simulink model "ROBOT_MODEL_5_OTT"  (R2020a)
settings: Solver=FixedStepAuto  StartTime=0.0  StopTime=3  FixedStep=0.0001  RelTol=1e-3
values from neighbouring files (symbols this model uses):
  g = 9.81    [fast_init.m]
  I1 = 1    [fast_init.m]
  I2 = 10    [fast_init.m]
  ini_theta1 = 0    [fast_init.m]
  ini_theta1_d = 0    [fast_init.m]
  ini_theta2 = 0    [fast_init.m]
  ini_theta2_d = 0    [fast_init.m]
  ini_x1 = ini_x0+r1*cos(pi/2 - ini_theta1)    [fast_init.m]
  ini_x1_d = 0    [fast_init.m]
  ini_x2 = ini_xH + r2*cos(pi/2 - ini_theta2)    [fast_init.m]
  ini_x2_d = 0    [fast_init.m]
  ini_y1 = ini_y0+r1*sin(pi/2 - ini_theta1)    [fast_init.m]
  ini_y1_d = 0    [fast_init.m]
  M1 = 1    [fast_init.m]
  M2 = 10    [fast_init.m]
  r1 = 0.5    [fast_init.m]
  r2 = 0.4    [fast_init.m]
settings Model: Creator=fabia  LastModifiedBy=mic-ciciolla

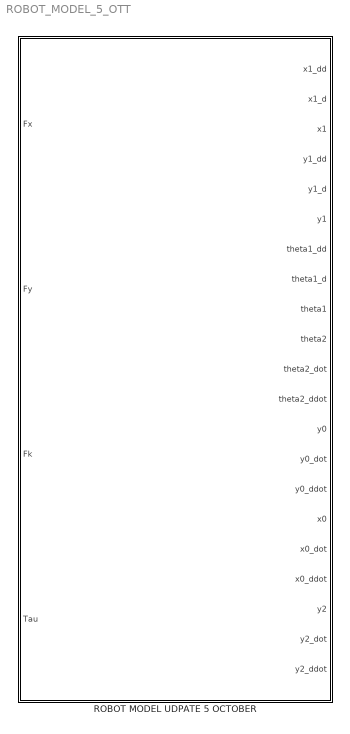
== system ROBOT_MODEL_5_OTT ==
  " ROBOT MODEL UDPATE 5 OCTOBER " : Subsystem

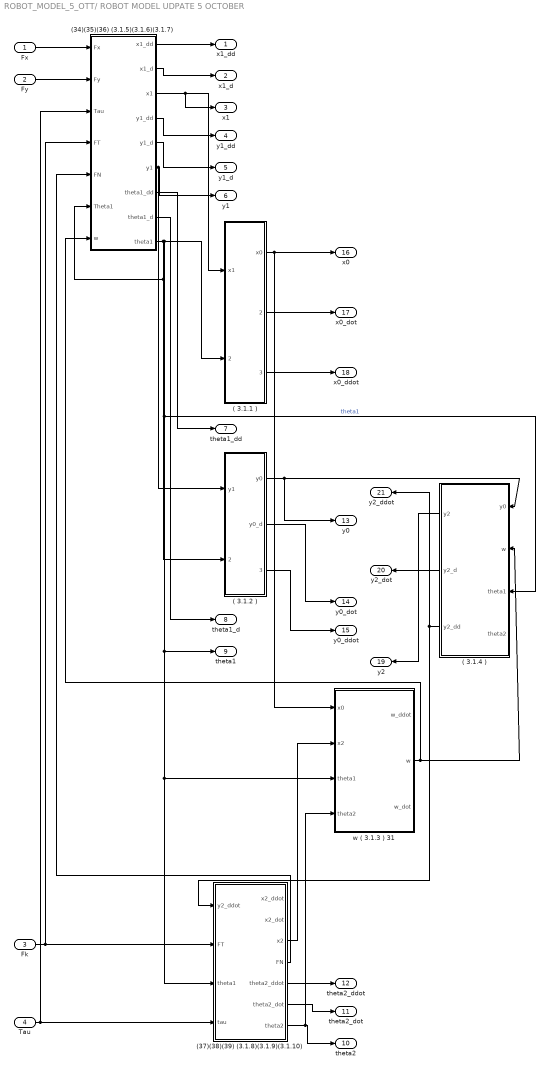
== system ROBOT_MODEL_5_OTT/ ROBOT MODEL UDPATE 5 OCTOBER  ==
  Fx : Inport
  Fy : Inport  Port=2
  Fk : Inport  Port=3
  Tau : Inport  Port=4
  "( 3.1.1 ) " : Subsystem
  ( 3.1.2 ) : Subsystem
  ( 3.1.4 ) : Subsystem
  (34)(35)(36) (3.1.5)(3.1.6)(3.1.7) : Subsystem
  (37)(38)(39) (3.1.8)(3.1.9)(3.1.10) : Subsystem
  w ( 3.1.3 ) 31 : Subsystem
  x1_dd : Outport
  x1_d : Outport  Port=2
  x1 : Outport  Port=3
  y1_dd : Outport  Port=4
  y1_d : Outport  Port=5
  y1 : Outport  Port=6
  theta1_dd : Outport  Port=7
  theta1_d : Outport  Port=8
  theta1 : Outport  Port=9
  theta2 : Outport  Port=10
  theta2_dot : Outport  Port=11
  theta2_ddot : Outport  Port=12
  y0 : Outport  Port=13
  y0_dot : Outport  Port=14
  y0_ddot : Outport  Port=15
  x0 : Outport  Port=16
  x0_dot : Outport  Port=17
  x0_ddot : Outport  Port=18
  y2 : Outport  Port=19
  y2_dot : Outport  Port=20
  y2_ddot : Outport  Port=21
  wires:
  ( 3.1.2 )/1(y0) -> ( 3.1.4 )/1(y0), y0/1
  "( 3.1.1 ) "/1(x0) -> w ( 3.1.3 ) 31/1(x0), x0/1
  ( 3.1.4 )/3(y2_dd) -> (37)(38)(39) (3.1.8)(3.1.9)(3.1.10)/1(y2_ddot), y2_ddot/1
  (34)(35)(36) (3.1.5)(3.1.6)(3.1.7)/3(x1) -> "( 3.1.1 ) "/1(x1), x1/1
  ( 3.1.4 )/2(y2_d) -> y2_dot/1
  (34)(35)(36) (3.1.5)(3.1.6)(3.1.7)/4(y1_dd) -> y1_dd/1
  ( 3.1.2 )/3(y0_dd) -> y0_ddot/1
  (37)(38)(39) (3.1.8)(3.1.9)(3.1.10)/3(x2) -> w ( 3.1.3 ) 31/2(x2)
  (37)(38)(39) (3.1.8)(3.1.9)(3.1.10)/4(FN) -> (34)(35)(36) (3.1.5)(3.1.6)(3.1.7)/5(FN)
  (34)(35)(36) (3.1.5)(3.1.6)(3.1.7)/1(x1_dd) -> x1_dd/1
  (37)(38)(39) (3.1.8)(3.1.9)(3.1.10)/5(theta2_ddot) -> theta2_ddot/1
  w ( 3.1.3 ) 31/2(w) -> ( 3.1.4 )/2(w), (34)(35)(36) (3.1.5)(3.1.6)(3.1.7)/7(w)
  (37)(38)(39) (3.1.8)(3.1.9)(3.1.10)/6(theta2_dot) -> theta2_dot/1
  Fy/1 -> (34)(35)(36) (3.1.5)(3.1.6)(3.1.7)/2(Fy)
  ( 3.1.4 )/1(y2) -> y2/1
  (37)(38)(39) (3.1.8)(3.1.9)(3.1.10)/7(theta2) -> w ( 3.1.3 ) 31/4(theta2), theta2/1
  (34)(35)(36) (3.1.5)(3.1.6)(3.1.7)/7(theta1_dd) -> theta1_dd/1
  Fx/1 -> (34)(35)(36) (3.1.5)(3.1.6)(3.1.7)/1(Fx)
  (34)(35)(36) (3.1.5)(3.1.6)(3.1.7)/2(x1_d) -> x1_d/1
  "( 3.1.1 ) "/2(x0_dot) -> x0_dot/1
  ( 3.1.2 )/2(y0_d) -> y0_dot/1
  Tau/1 -> (34)(35)(36) (3.1.5)(3.1.6)(3.1.7)/3(Tau), (37)(38)(39) (3.1.8)(3.1.9)(3.1.10)/4(tau)
  (34)(35)(36) (3.1.5)(3.1.6)(3.1.7)/8(theta1_d) -> theta1_d/1
  (34)(35)(36) (3.1.5)(3.1.6)(3.1.7)/5(y1_d) -> y1_d/1
  "( 3.1.1 ) "/3(x0_ddot) -> x0_ddot/1
  (34)(35)(36) (3.1.5)(3.1.6)(3.1.7)/6(y1) -> ( 3.1.2 )/1(y1), y1/1
  (34)(35)(36) (3.1.5)(3.1.6)(3.1.7)/9(theta1) -> ( 3.1.2 )/2(theta1), (34)(35)(36) (3.1.5)(3.1.6)(3.1.7)/6(Theta1), (37)(38)(39) (3.1.8)(3.1.9)(3.1.10)/3(theta1), w ( 3.1.3 ) 31/3(theta1), theta1/1, ( 3.1.4 )/3(theta1), "( 3.1.1 ) "/2(theta1)  "theta1"
  Fk/1 -> (34)(35)(36) (3.1.5)(3.1.6)(3.1.7)/4(FT), (37)(38)(39) (3.1.8)(3.1.9)(3.1.10)/2(FT)

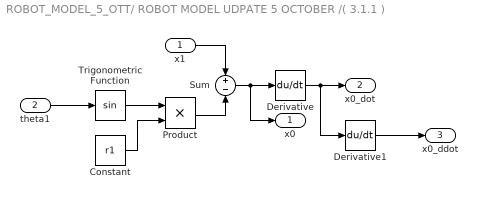
== system ROBOT_MODEL_5_OTT/ ROBOT MODEL UDPATE 5 OCTOBER /( 3.1.1 )  ==
  x1 : Inport
  theta1 : Inport  Port=2
  Constant : Constant  Value=r1
  Derivative : Derivative
  Derivative1 : Derivative
  Product : Product
  Sum : Sum  Inputs=+-
  Trigonometric Function : Trigonometry
  x0 : Outport
  x0_dot : Outport  Port=2
  x0_ddot : Outport  Port=3
  wires:
  Sum/1 -> x0/1, Derivative/1
  Derivative/1 -> x0_dot/1, Derivative1/1
  theta1/1 -> Trigonometric Function/1
  Trigonometric Function/1 -> Product/1
  x1/1 -> Sum/1
  Product/1 -> Sum/2
  Derivative1/1 -> x0_ddot/1
  Constant/1 -> Product/2

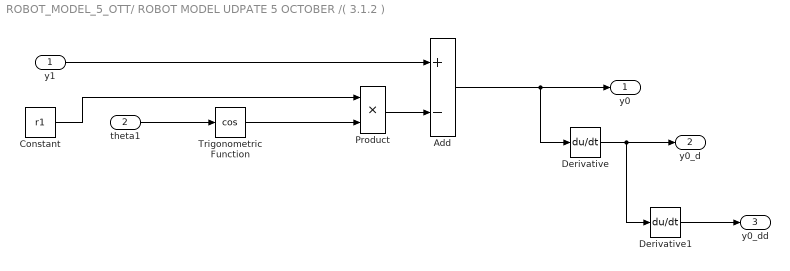
== system ROBOT_MODEL_5_OTT/ ROBOT MODEL UDPATE 5 OCTOBER /( 3.1.2 ) ==
  y1 : Inport
  theta1 : Inport  Port=2
  Add : Sum  Inputs=+-
  Constant : Constant  Value=r1
  Derivative : Derivative
  Derivative1 : Derivative
  Product : Product
  Trigonometric Function : Trigonometry  Operator=cos
  y0 : Outport
  y0_d : Outport  Port=2
  y0_dd : Outport  Port=3
  wires:
  y1/1 -> Add/1
  theta1/1 -> Trigonometric Function/1
  Trigonometric Function/1 -> Product/2
  Add/1 -> Derivative/1, y0/1
  Derivative/1 -> y0_d/1, Derivative1/1
  Derivative1/1 -> y0_dd/1
  Product/1 -> Add/2
  Constant/1 -> Product/1

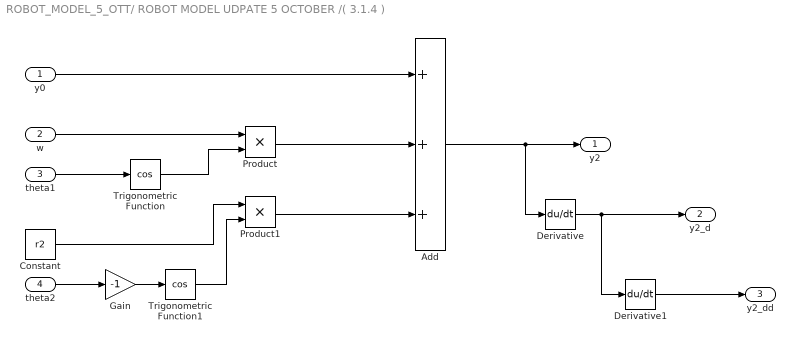
== system ROBOT_MODEL_5_OTT/ ROBOT MODEL UDPATE 5 OCTOBER /( 3.1.4 ) ==
  y0 : Inport
  w : Inport  Port=2
  theta1 : Inport  Port=3
  theta2 : Inport  Port=4
  Add : Sum  Inputs=+++
  Constant : Constant  Value=r2
  Derivative : Derivative
  Derivative1 : Derivative
  Gain : Gain  Gain=-1
  Product : Product
  Product1 : Product
  Trigonometric Function : Trigonometry  Operator=cos
  Trigonometric Function1 : Trigonometry  Operator=cos
  y2 : Outport
  y2_d : Outport  Port=2
  y2_dd : Outport  Port=3
  wires:
  y0/1 -> Add/1
  theta1/1 -> Trigonometric Function/1
  w/1 -> Product/1
  Trigonometric Function/1 -> Product/2
  Product/1 -> Add/2
  theta2/1 -> Gain/1
  Gain/1 -> Trigonometric Function1/1
  Trigonometric Function1/1 -> Product1/2
  Constant/1 -> Product1/1
  Product1/1 -> Add/3
  Add/1 -> Derivative/1, y2/1
  Derivative/1 -> y2_d/1, Derivative1/1
  Derivative1/1 -> y2_dd/1

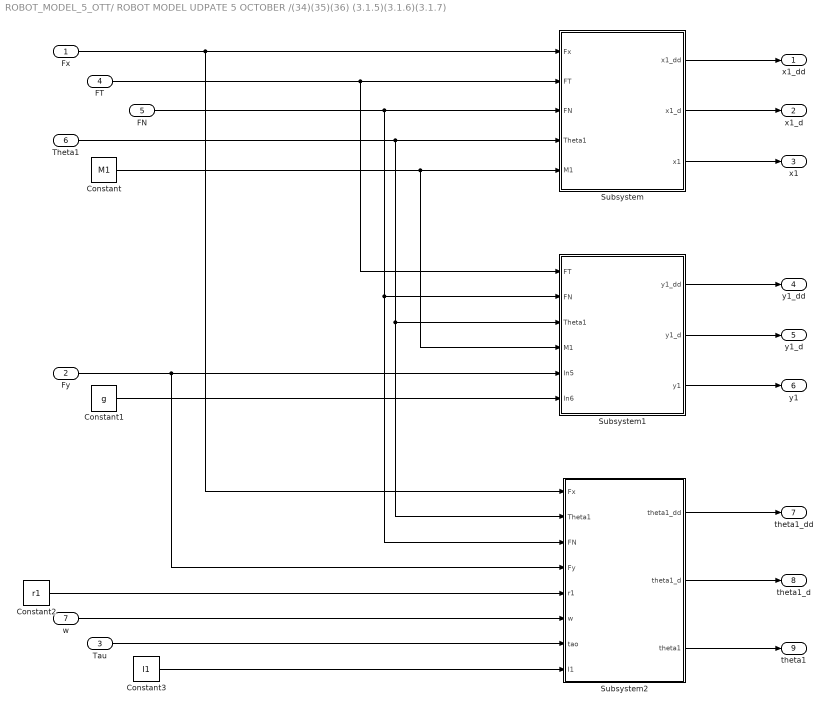
== system ROBOT_MODEL_5_OTT/ ROBOT MODEL UDPATE 5 OCTOBER /(34)(35)(36) (3.1.5)(3.1.6)(3.1.7) ==
  Fx : Inport
  Fy : Inport  Port=2
  Tau : Inport  Port=3
  FT : Inport  Port=4
  FN : Inport  Port=5
  Theta1 : Inport  Port=6
  w : Inport  Port=7
  Constant : Constant  Value=M1
  Constant1 : Constant  Value=g
  Constant2 : Constant  Value=r1
  Constant3 : Constant  Value=I1
  Subsystem : Subsystem
  Subsystem1 : Subsystem
  Subsystem2 : Subsystem
  x1_dd : Outport
  x1_d : Outport  Port=2
  x1 : Outport  Port=3
  y1_dd : Outport  Port=4
  y1_d : Outport  Port=5
  y1 : Outport  Port=6
  theta1_dd : Outport  Port=7
  theta1_d : Outport  Port=8
  theta1 : Outport  Port=9
  wires:
  Subsystem1/2(y1_d) -> y1_d/1
  Subsystem2/2(theta1_d) -> theta1_d/1
  Constant2/1 -> Subsystem2/5(r1)
  Subsystem/3(x1) -> x1/1
  Subsystem/2(x1_d) -> x1_d/1
  Subsystem1/1(y1_dd) -> y1_dd/1
  Constant1/1 -> Subsystem1/6(In6)
  Theta1/1 -> Subsystem2/2(Theta1), Subsystem1/3(Theta1), Subsystem/4(Theta1)
  Subsystem2/1(theta1_dd) -> theta1_dd/1
  Fx/1 -> Subsystem/1(Fx), Subsystem2/1(Fx)
  Subsystem1/3(y1) -> y1/1
  Subsystem2/3(theta1) -> theta1/1
  FN/1 -> Subsystem2/3(FN), Subsystem1/2(FN), Subsystem/3(FN)
  Tau/1 -> Subsystem2/7(tao)
  Subsystem/1(x1_dd) -> x1_dd/1
  Fy/1 -> Subsystem1/5(In5), Subsystem2/4(Fy)
  FT/1 -> Subsystem/2(FT), Subsystem1/1(FT)
  w/1 -> Subsystem2/6(w)
  Constant/1 -> Subsystem1/4(M1), Subsystem/5(M1)
  Constant3/1 -> Subsystem2/8(I1)

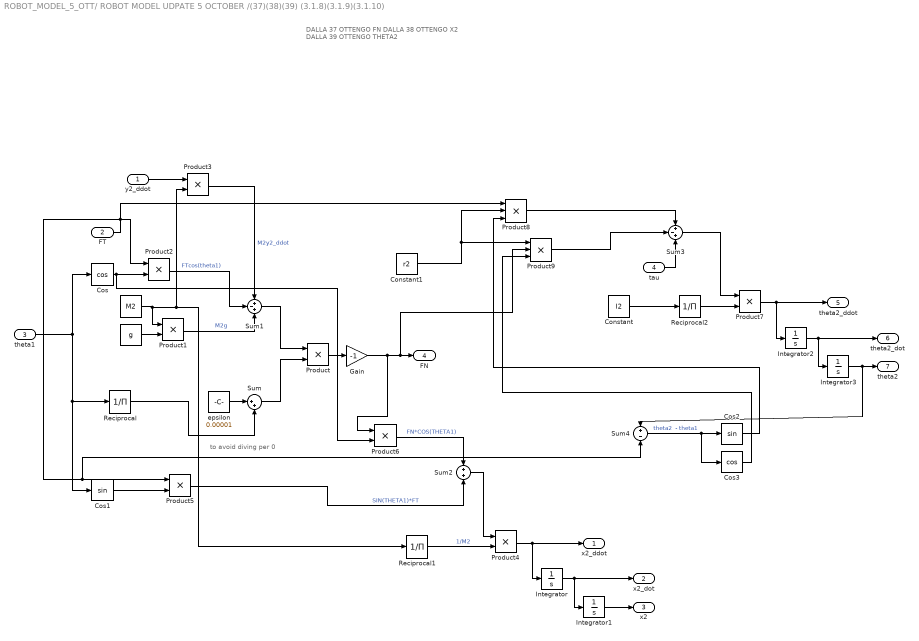
== system ROBOT_MODEL_5_OTT/ ROBOT MODEL UDPATE 5 OCTOBER /(37)(38)(39) (3.1.8)(3.1.9)(3.1.10) ==
  note: to avoid diving per 0
  note: DALLA 37 OTTENGO FN
      | DALLA 38 OTTENGO X2
      | DALLA 39 OTTENGO THETA2
  y2_ddot : Inport
  FT : Inport  Port=2
  theta1 : Inport  Port=3
  tau : Inport  Port=4
  " " : Constant  Value=M2
  "  " : Constant  Value=g
  Constant : Constant  Value=I2
  Constant1 : Constant  Value=r2
  Cos : Trigonometry  Operator=cos
  Cos1 : Trigonometry
  Cos2 : Trigonometry
  Cos3 : Trigonometry  Operator=cos
  Gain : Gain  Gain=-1
  Integrator : Integrator  InitialCondition=ini_x2_d
  Integrator1 : Integrator  InitialCondition=ini_x2
  Integrator2 : Integrator  InitialCondition=ini_theta2_d
  Integrator3 : Integrator  InitialCondition=ini_theta2
  Product{,1..7} (8 alike) : Product
  Product8 : Product  Inputs=3
  Product9 : Product  Inputs=3
  Reciprocal : Product  Inputs=/
  Reciprocal1 : Product  Inputs=/
  Reciprocal2 : Product  Inputs=/
  Sum : Sum  Inputs=|++
  Sum1 : Sum  Inputs=+-+
  Sum2 : Sum
  Sum3 : Sum  Inputs=+-+
  Sum4 : Sum  Inputs=+-
  epsilon : Constant  Value=0.00001
  x2_ddot : Outport
  x2_dot : Outport  Port=2
  x2 : Outport  Port=3
  FN : Outport  Port=4
  theta2_ddot : Outport  Port=5
  theta2_dot : Outport  Port=6
  theta2 : Outport  Port=7
  wires:
  theta1/1 -> Cos/1, Cos1/1, Reciprocal/1
  Gain/1 -> Product6/1, Product9/2, FN/1
  Product/1 -> Gain/1
  Reciprocal/1 -> Sum/2
  Sum/1 -> Product/2
  epsilon/1 -> Sum/1
  "  "/1 -> Product1/2
  " "/1 -> Reciprocal1/1, Product3/2, Product1/1
  Product1/1 -> Sum1/3  "M2g"
  Cos/1 -> Product6/2, Product2/2
  FT/1 -> Product8/1, Product2/1, Sum4/2, Product5/1
  Product2/1 -> Sum1/2  "FTcos(theta1)"
  y2_ddot/1 -> Product3/1
  Product3/1 -> Sum1/1  "M2y2_ddot"
  Sum1/1 -> Product/1
  Product4/1 -> Integrator/1, x2_ddot/1
  Reciprocal1/1 -> Product4/2  "1/M2"
  Sum2/1 -> Product4/1
  Cos1/1 -> Product5/2
  Product6/1 -> Sum2/1  "FN*COS(THETA1)"
  Product5/1 -> Sum2/2  "SIN(THETA1)*FT"
  Integrator/1 -> Integrator1/1, x2_dot/1
  Integrator1/1 -> x2/1
  Constant/1 -> Reciprocal2/1
  Reciprocal2/1 -> Product7/2
  Sum3/1 -> Product7/1
  Product7/1 -> Integrator2/1, theta2_ddot/1
  Integrator2/1 -> Integrator3/1, theta2_dot/1
  Integrator3/1 -> theta2/1, Sum4/1
  tau/1 -> Sum3/3
  Sum4/1 -> Cos3/1, Cos2/1  "theta2  - theta1"
  Constant1/1 -> Product9/1, Product8/2
  Cos2/1 -> Product8/3
  Product8/1 -> Sum3/1
  Product9/1 -> Sum3/2
  Cos3/1 -> Product9/3

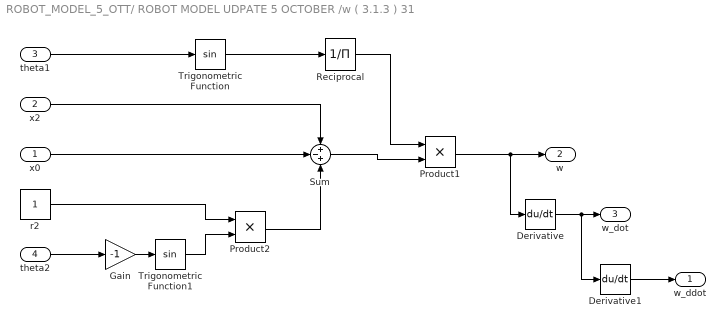
== system ROBOT_MODEL_5_OTT/ ROBOT MODEL UDPATE 5 OCTOBER /w ( 3.1.3 ) 31 ==
  x0 : Inport
  x2 : Inport  Port=2
  theta1 : Inport  Port=3
  theta2 : Inport  Port=4
  Derivative : Derivative
  Derivative1 : Derivative
  Gain : Gain  Gain=-1
  Product1 : Product
  Product2 : Product
  Reciprocal : Product  Inputs=/
  Sum : Sum  Inputs=+-+
  Trigonometric Function : Trigonometry
  Trigonometric Function1 : Trigonometry
  r2 : Constant
  w_ddot : Outport
  w : Outport  Port=2
  w_dot : Outport  Port=3
  wires:
  r2/1 -> Product2/1
  Trigonometric Function1/1 -> Product2/2
  Gain/1 -> Trigonometric Function1/1
  theta2/1 -> Gain/1
  Product2/1 -> Sum/3
  Sum/1 -> Product1/2
  Derivative/1 -> Derivative1/1, w_dot/1
  Derivative1/1 -> w_ddot/1
  x2/1 -> Sum/1
  x0/1 -> Sum/2
  theta1/1 -> Trigonometric Function/1
  Trigonometric Function/1 -> Reciprocal/1
  Product1/1 -> Derivative/1, w/1
  Reciprocal/1 -> Product1/1

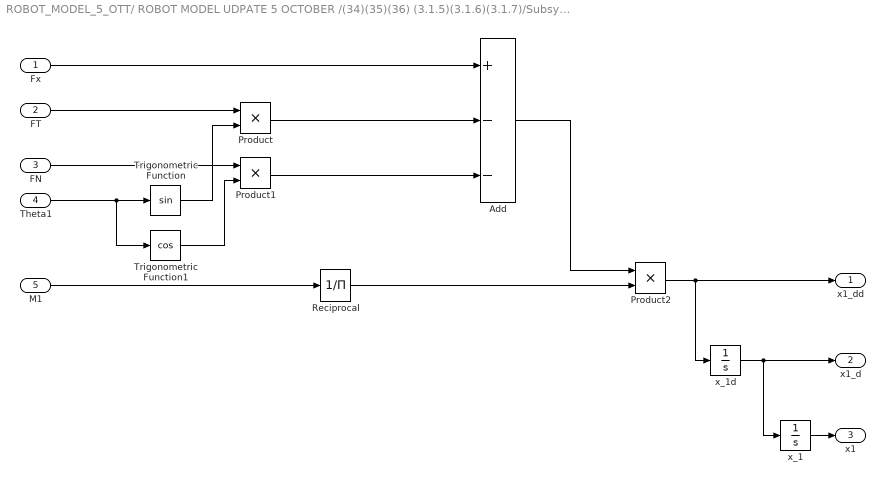
== system ROBOT_MODEL_5_OTT/ ROBOT MODEL UDPATE 5 OCTOBER /(34)(35)(36) (3.1.5)(3.1.6)(3.1.7)/Subsystem ==
  Fx : Inport
  FT : Inport  Port=2
  FN : Inport  Port=3
  Theta1 : Inport  Port=4
  M1 : Inport  Port=5
  Add : Sum  Inputs=+--
  Product : Product
  Product1 : Product
  Product2 : Product
  Reciprocal : Product  Inputs=/
  Trigonometric Function : Trigonometry
  Trigonometric Function1 : Trigonometry  Operator=cos
  x_1 : Integrator  InitialCondition=ini_x1
  x_1d : Integrator  InitialCondition=ini_x1_d
  x1_dd : Outport
  x1_d : Outport  Port=2
  x1 : Outport  Port=3
  wires:
  Add/1 -> Product2/1
  FN/1 -> Product1/1
  Reciprocal/1 -> Product2/2
  Trigonometric Function1/1 -> Product1/2
  Theta1/1 -> Trigonometric Function/1, Trigonometric Function1/1
  Product1/1 -> Add/3
  Trigonometric Function/1 -> Product/2
  Product2/1 -> x_1d/1, x1_dd/1
  Product/1 -> Add/2
  FT/1 -> Product/1
  Fx/1 -> Add/1
  M1/1 -> Reciprocal/1
  x_1d/1 -> x_1/1, x1_d/1
  x_1/1 -> x1/1

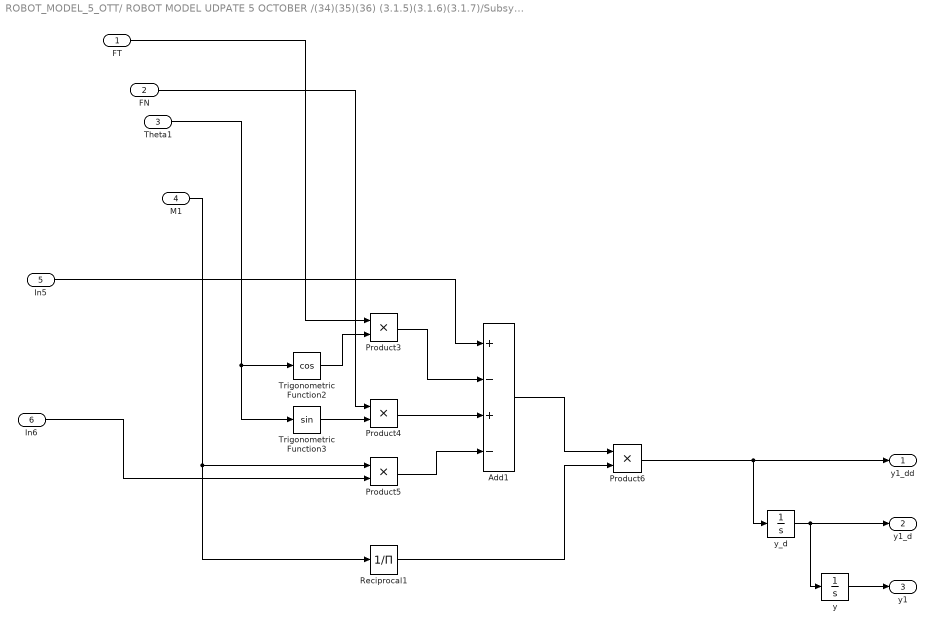
== system ROBOT_MODEL_5_OTT/ ROBOT MODEL UDPATE 5 OCTOBER /(34)(35)(36) (3.1.5)(3.1.6)(3.1.7)/Subsystem1 ==
  FT : Inport
  FN : Inport  Port=2
  Theta1 : Inport  Port=3
  M1 : Inport  Port=4
  In5 : Inport  Port=5
  In6 : Inport  Port=6
  Add1 : Sum  Inputs=+-+-
  Product{3..6} (4 alike) : Product
  Reciprocal1 : Product  Inputs=/
  Trigonometric Function2 : Trigonometry  Operator=cos
  Trigonometric Function3 : Trigonometry
  y : Integrator  InitialCondition=ini_y1
  y_d : Integrator  InitialCondition=ini_y1_d
  y1_dd : Outport
  y1_d : Outport  Port=2
  y1 : Outport  Port=3
  wires:
  Product3/1 -> Add1/2
  Product4/1 -> Add1/3
  Theta1/1 -> Trigonometric Function2/1, Trigonometric Function3/1
  M1/1 -> Product5/1, Reciprocal1/1
  Trigonometric Function3/1 -> Product4/2
  Trigonometric Function2/1 -> Product3/2
  Reciprocal1/1 -> Product6/2
  Product5/1 -> Add1/4
  Add1/1 -> Product6/1
  In5/1 -> Add1/1
  In6/1 -> Product5/2
  FT/1 -> Product3/1
  FN/1 -> Product4/1
  Product6/1 -> y_d/1, y1_dd/1
  y_d/1 -> y/1, y1_d/1
  y/1 -> y1/1

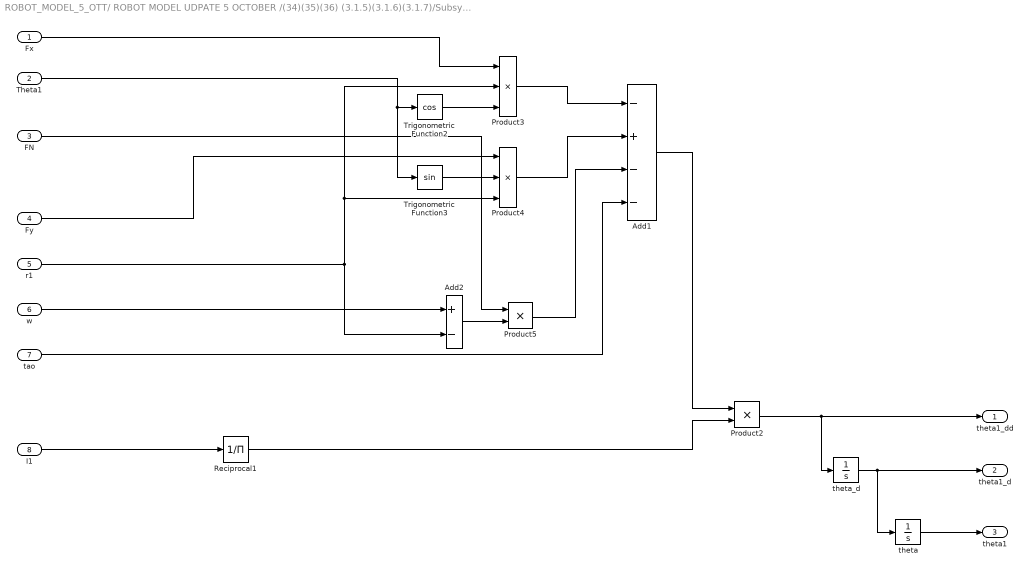
== system ROBOT_MODEL_5_OTT/ ROBOT MODEL UDPATE 5 OCTOBER /(34)(35)(36) (3.1.5)(3.1.6)(3.1.7)/Subsystem2 ==
  Fx : Inport
  Theta1 : Inport  Port=2
  FN : Inport  Port=3
  Fy : Inport  Port=4
  r1 : Inport  Port=5
  w : Inport  Port=6
  tao : Inport  Port=7
  I1 : Inport  Port=8
  Add1 : Sum  Inputs=-+--
  Add2 : Sum  Inputs=+-
  Product2 : Product
  Product3 : Product  Inputs=3
  Product4 : Product  Inputs=3
  Product5 : Product
  Reciprocal1 : Product  Inputs=/
  Trigonometric Function2 : Trigonometry  Operator=cos
  Trigonometric Function3 : Trigonometry
  theta : Integrator  InitialCondition=ini_theta1
  theta_d : Integrator  InitialCondition=ini_theta1_d
  theta1_dd : Outport
  theta1_d : Outport  Port=2
  theta1 : Outport  Port=3
  wires:
  Product5/1 -> Add1/3
  r1/1 -> Product3/2, Product4/3, Add2/2
  Trigonometric Function2/1 -> Product3/3
  Reciprocal1/1 -> Product2/2
  Product2/1 -> theta_d/1, theta1_dd/1
  Add1/1 -> Product2/1
  Add2/1 -> Product5/2
  Product4/1 -> Add1/2
  Theta1/1 -> Trigonometric Function3/1, Trigonometric Function2/1
  Trigonometric Function3/1 -> Product4/2
  Product3/1 -> Add1/1
  Fx/1 -> Product3/1
  tao/1 -> Add1/4
  I1/1 -> Reciprocal1/1
  Fy/1 -> Product4/1
  FN/1 -> Product5/1
  w/1 -> Add2/1
  theta_d/1 -> theta1_d/1, theta/1
  theta/1 -> theta1/1
